simulink model "LGS_allFaultStuffDeleted"  (R2019b)
settings: Solver=FixedStepDiscrete  StartTime=0.0  StopTime=45.0  FixedStep=0.1  RelTol=1e-3
model workspace (MAT data in the model file):
  fipData : object (value not decoded)
  fipName : object (value not decoded)
  stepSize = 0.1
libraries: commrandsrc3 x16, simulink x3, LibFailureCondition x1
(part 2 of 7)

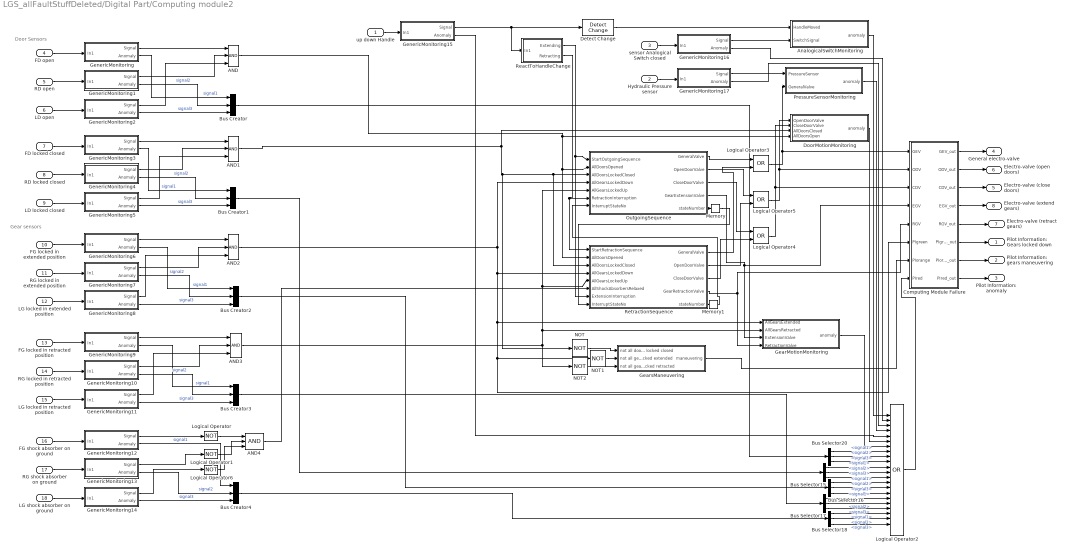
== system LGS_allFaultStuffDeleted/Digital Part/Computing module2 ==
  note: Gear sensors
  note: Door Sensors
  up down Handle : Inport
  Hydraulic Pressure sensor : Inport  Port=2
  " sensor Analogical Switch closed" : Inport  Port=3
  FD open : Inport  Port=4
  RD open : Inport  Port=5
  LD open : Inport  Port=6
  FD locked closed : Inport  Port=7
  RD locked closed : Inport  Port=8
  LD locked closed : Inport  Port=9
  FG locked in extended position : Inport  Port=10
  RG locked in extended position : Inport  Port=11
  LG locked in extended position : Inport  Port=12
  FG locked in retracted position : Inport  Port=13
  RG locked in retracted position : Inport  Port=14
  LG locked in retracted position : Inport  Port=15
  FG shock absorber on ground : Inport  Port=16
  RG shock absorber on ground : Inport  Port=17
  LG shock absorber on ground : Inport  Port=18
  AND{,1..4} (5 alike) : Logic  Inputs=3  IconShape=distinctive  AllPortsSameDT=off  OutDataTypeStr=boolean
  AnalogicalSwitchMonitoring : Stateflow chart  TreatAsAtomicUnit=on
  Bus Creator{,1..4} (5 alike) : BusCreator  Inputs=3
  Bus Selector{15..18,20} (5 alike) : BusSelector  OutputSignals=signal1,signal2,signal3
  Computing Module Failure : Subsystem
  Detect Change : simulink/Logic and Bit Operations/Detect Change  vinit=1  OutDataTypeStr=boolean
  DoorMotionMonitoring : Stateflow chart  TreatAsAtomicUnit=on
  GearMotionMonitoring : Stateflow chart  TreatAsAtomicUnit=on
  GearsManeuvering : Subsystem
  GenericMonitoring : Subsystem
  GenericMonitoring1 : Subsystem
  GenericMonitoring10 : Subsystem
  GenericMonitoring11 : Subsystem
  GenericMonitoring12 : Subsystem
  GenericMonitoring13 : Subsystem
  GenericMonitoring14 : Subsystem
  GenericMonitoring15 : Subsystem
  GenericMonitoring16 : Subsystem
  GenericMonitoring17 : Subsystem
  GenericMonitoring2 : Subsystem
  GenericMonitoring3 : Subsystem
  GenericMonitoring4 : Subsystem
  GenericMonitoring5 : Subsystem
  GenericMonitoring6 : Subsystem
  GenericMonitoring7 : Subsystem
  GenericMonitoring8 : Subsystem
  GenericMonitoring9 : Subsystem
  Logical Operator : Logic  Operator=NOT  AllPortsSameDT=off  OutDataTypeStr=boolean
  Logical Operator1 : Logic  Operator=NOT  AllPortsSameDT=off  OutDataTypeStr=boolean
  Logical Operator2 : Logic  Operator=OR  Inputs=22  AllPortsSameDT=off  OutDataTypeStr=boolean
  Logical Operator3 : Logic  Operator=OR  AllPortsSameDT=off  OutDataTypeStr=boolean
  Logical Operator4 : Logic  Operator=OR  AllPortsSameDT=off  OutDataTypeStr=boolean
  Logical Operator5 : Logic  Operator=OR  AllPortsSameDT=off  OutDataTypeStr=boolean
  Logical Operator6 : Logic  Operator=NOT  AllPortsSameDT=off  OutDataTypeStr=boolean
  Memory : Memory  InheritSampleTime=on
  Memory1 : Memory  InheritSampleTime=on
  NOT : Logic  Operator=NOT  IconShape=distinctive  AllPortsSameDT=off  OutDataTypeStr=boolean
  NOT1 : Logic  Operator=NOT  IconShape=distinctive  AllPortsSameDT=off  OutDataTypeStr=boolean
  NOT2 : Logic  Operator=NOT  IconShape=distinctive  AllPortsSameDT=off  OutDataTypeStr=boolean
  OutgoingSequence : Stateflow chart  TreatAsAtomicUnit=on
  PressureSensorMonitoring : Stateflow chart  TreatAsAtomicUnit=on
  ReactToHandleChange : Subsystem
  RetractionSequence : Stateflow chart  TreatAsAtomicUnit=on
  Pilot Information: Gears locked down : Outport  OutDataTypeStr=boolean
  Pilot Information: gears maneuvering : Outport  Port=2  OutDataTypeStr=boolean
  Pilot Information: anomaly : Outport  Port=3  OutDataTypeStr=boolean
  General electro-valve : Outport  Port=4
  Electro-valve (close doors) : Outport  Port=5
  Electro-valve (open doors) : Outport  Port=6
  Electro-valve (retract gears) : Outport  Port=7
  Electro-valve (extend gears) : Outport  Port=8
  wires:
  ReactToHandleChange/1(Extending) -> RetractionSequence/7(ExtensionInterruption), OutgoingSequence/1(StartOutgoingSequence)
  OutgoingSequence/1(GeneralValve) -> Logical Operator3/1
  OutgoingSequence/2(OpenDoorValve) -> Logical Operator5/1
  OutgoingSequence/4(GearExtensionValve) -> Computing Module Failure/4(EGV), GearMotionMonitoring/3(ExtensionValve)
  OutgoingSequence/3(CloseDoorValve) -> Logical Operator4/1
  FD open/1 -> GenericMonitoring/1(In1)
  RD open/1 -> GenericMonitoring1/1(In1)
  LD open/1 -> GenericMonitoring2/1(In1)
  AND/1 -> DoorMotionMonitoring/4(AllDoorsOpen), RetractionSequence/2(AllDoorsOpened), OutgoingSequence/2(AllDoorsOpened)
  FD locked closed/1 -> GenericMonitoring3/1(In1)
  RD locked closed/1 -> GenericMonitoring4/1(In1)
  LD locked closed/1 -> GenericMonitoring5/1(In1)
  AND1/1 -> NOT/1, RetractionSequence/3(AllDoorsLockedClosed), OutgoingSequence/3(AllDoorsLockedClosed), DoorMotionMonitoring/3(AllDoorsClosed)
  FG locked in extended position/1 -> GenericMonitoring6/1(In1)
  RG locked in extended position/1 -> GenericMonitoring7/1(In1)
  LG locked in extended position/1 -> GenericMonitoring8/1(In1)
  FG locked in retracted position/1 -> GenericMonitoring9/1(In1)
  RG locked in retracted position/1 -> GenericMonitoring10/1(In1)
  LG locked in retracted position/1 -> GenericMonitoring11/1(In1)
  LG shock absorber on ground/1 -> GenericMonitoring14/1(In1)
  AND2/1 -> Computing Module Failure/6(PIgreen), NOT1/1, GearMotionMonitoring/1(AllGearsExtended), RetractionSequence/4(AllGearsLockedDown), OutgoingSequence/4(AllGearsLockedDown)
  GearsManeuvering/1(maneuvering) -> Computing Module Failure/7(PIorange)
  FG shock absorber on ground/1 -> GenericMonitoring12/1(In1)
  GenericMonitoring12/1(Signal) -> Logical Operator/1
  GenericMonitoring13/1(Signal) -> Logical Operator1/1
  GenericMonitoring14/1(Signal) -> Logical Operator6/1
  AnalogicalSwitchMonitoring/1(anomaly) -> Logical Operator2/1
  Detect Change/1 -> AnalogicalSwitchMonitoring/1(HandleMoved)
  " sensor Analogical Switch closed"/1 -> GenericMonitoring16/1(In1)
  Hydraulic Pressure sensor/1 -> GenericMonitoring17/1(In1)
  PressureSensorMonitoring/1(anomaly) -> Logical Operator2/4
  DoorMotionMonitoring/1(anomaly) -> Logical Operator2/6
  GearMotionMonitoring/1(anomaly) -> Logical Operator2/7
  Logical Operator2/1 -> Computing Module Failure/8(PIred)
  RG shock absorber on ground/1 -> GenericMonitoring13/1(In1)
  RetractionSequence/1(GeneralValve) -> Logical Operator3/2
  Logical Operator3/1 -> Computing Module Failure/1(GEV), PressureSensorMonitoring/2(GeneralValve)
  RetractionSequence/3(CloseDoorValve) -> Logical Operator4/2
  Logical Operator4/1 -> Computing Module Failure/3(CDV), DoorMotionMonitoring/2(CloseDoorValve)
  RetractionSequence/2(OpenDoorValve) -> Logical Operator5/2
  Logical Operator5/1 -> Computing Module Failure/2(ODV), DoorMotionMonitoring/1(OpenDoorValve)
  RetractionSequence/4(GearRetractionValve) -> Computing Module Failure/5(RGV), GearMotionMonitoring/4(RetractionValve)
  GenericMonitoring/2(Anomaly) -> Bus Creator/1  "signal1"
  GenericMonitoring2/2(Anomaly) -> Bus Creator/3  "signal3"
  GenericMonitoring1/2(Anomaly) -> Bus Creator/2  "signal2"
  Bus Creator/1 -> Bus Selector20/1
  AND3/1 -> GearMotionMonitoring/2(AllGearsRetracted), RetractionSequence/5(AllGearsLockedUp), OutgoingSequence/5(AllGearsLockedUp), NOT2/1
  ReactToHandleChange/2(Retracting) -> RetractionSequence/1(StartRetractionSequence), OutgoingSequence/6(RetractionInterruption)
  Bus Selector15/1 -> Logical Operator2/11  "<signal1>"
  Bus Selector15/2 -> Logical Operator2/12  "<signal2>"
  Bus Selector15/3 -> Logical Operator2/13  "<signal3>"
  Bus Selector16/1 -> Logical Operator2/14  "<signal1>"
  Bus Selector16/2 -> Logical Operator2/15  "<signal2>"
  Bus Selector16/3 -> Logical Operator2/16  "<signal3>"
  Bus Selector17/1 -> Logical Operator2/17  "<signal1>"
  Bus Selector17/2 -> Logical Operator2/18  "<signal2>"
  Bus Selector17/3 -> Logical Operator2/19  "<signal3>"
  Bus Selector18/1 -> Logical Operator2/20  "<signal1>"
  Bus Selector18/2 -> Logical Operator2/21  "<signal2>"
  Bus Selector18/3 -> Logical Operator2/22  "<signal3>"
  Bus Selector20/1 -> Logical Operator2/8  "<signal1>"
  Bus Selector20/2 -> Logical Operator2/9  "<signal2>"
  Bus Selector20/3 -> Logical Operator2/10  "<signal3>"
  GenericMonitoring12/2(Anomaly) -> Bus Creator4/1  "signal1"
  GenericMonitoring3/2(Anomaly) -> Bus Creator1/1  "signal1"
  GenericMonitoring4/2(Anomaly) -> Bus Creator1/2  "signal2"
  GenericMonitoring5/2(Anomaly) -> Bus Creator1/3  "signal3"
  Bus Creator1/1 -> Bus Selector15/1
  GenericMonitoring8/2(Anomaly) -> Bus Creator2/3  "signal3"
  GenericMonitoring6/2(Anomaly) -> Bus Creator2/1  "signal1"
  GenericMonitoring7/2(Anomaly) -> Bus Creator2/2  "signal2"
  Bus Creator2/1 -> Bus Selector16/1
  GenericMonitoring11/2(Anomaly) -> Bus Creator3/3  "signal3"
  GenericMonitoring10/2(Anomaly) -> Bus Creator3/2  "signal2"
  GenericMonitoring9/2(Anomaly) -> Bus Creator3/1  "signal1"
  Bus Creator3/1 -> Bus Selector17/1
  GenericMonitoring13/2(Anomaly) -> Bus Creator4/2  "signal2"
  GenericMonitoring14/2(Anomaly) -> Bus Creator4/3  "signal3"
  Bus Creator4/1 -> Bus Selector18/1
  Logical Operator/1 -> AND4/1
  Logical Operator6/1 -> AND4/3
  GenericMonitoring17/1(Signal) -> PressureSensorMonitoring/1(PressureSensor)
  GenericMonitoring16/1(Signal) -> AnalogicalSwitchMonitoring/2(SwitchSignal)
  GenericMonitoring16/2(Anomaly) -> Logical Operator2/2
  up down Handle/1 -> GenericMonitoring15/1(In1)
  GenericMonitoring15/2(Anomaly) -> Logical Operator2/5
  GenericMonitoring17/2(Anomaly) -> Logical Operator2/3
  Memory/1 -> RetractionSequence/8(InterruptStateNo)
  Memory1/1 -> OutgoingSequence/7(InterruptStateNo)
  OutgoingSequence/5(stateNumber) -> Memory/1
  RetractionSequence/5(stateNumber) -> Memory1/1
  Computing Module Failure/1(GEV_out) -> General electro-valve/1
  Computing Module Failure/2(ODV_out) -> Electro-valve (open doors)/1
  Computing Module Failure/3(CDV_out) -> Electro-valve (close doors)/1
  Computing Module Failure/4(EGV_out) -> Electro-valve (extend gears)/1
  Computing Module Failure/5(RGV_out) -> Electro-valve (retract gears)/1
  Computing Module Failure/6(PIgreen_out) -> Pilot Information: Gears locked down/1
  Computing Module Failure/7(PIorange_out) -> Pilot Information: gears maneuvering/1
  Computing Module Failure/8(PIred_out) -> Pilot Information: anomaly/1
  AND4/1 -> RetractionSequence/6(AllShockAbsorbersRelaxed)
  GenericMonitoring15/1(Signal) -> Detect Change/1, ReactToHandleChange/1(In1)
  GenericMonitoring/1(Signal) -> AND/1
  GenericMonitoring1/1(Signal) -> AND/2
  GenericMonitoring2/1(Signal) -> AND/3
  GenericMonitoring3/1(Signal) -> AND1/1
  GenericMonitoring4/1(Signal) -> AND1/2
  GenericMonitoring5/1(Signal) -> AND1/3
  GenericMonitoring6/1(Signal) -> AND2/1
  GenericMonitoring7/1(Signal) -> AND2/2
  GenericMonitoring8/1(Signal) -> AND2/3
  GenericMonitoring9/1(Signal) -> AND3/1
  GenericMonitoring10/1(Signal) -> AND3/2
  GenericMonitoring11/1(Signal) -> AND3/3
  NOT/1 -> GearsManeuvering/1(not all doors locked closed)
  NOT1/1 -> GearsManeuvering/2(not all gears locked extended)
  NOT2/1 -> GearsManeuvering/3(not all gears locked retracted)
  Logical Operator1/1 -> AND4/2

== system LGS_allFaultStuffDeleted/Doors/EV close doors ==
  In1 : Inport
  In2 : Inport  Port=2
  Constant : Constant  Value=false  OutDataTypeStr=boolean
  EV close doors : Stateflow chart  TreatAsAtomicUnit=on
  Memory : Memory  InheritSampleTime=on
  Out1 : Outport
  wires:
  Memory/1 -> EV close doors/1(signal_in)
  In1/1 -> Memory/1
  In2/1 -> EV close doors/2(EVCloseDoorsPresure_in)
  EV close doors/1(EVCloseDoorsPresure_out) -> Out1/1
  Constant/1 -> EV close doors/3(fail)

== system LGS_allFaultStuffDeleted/Doors/EV open doors ==
  In1 : Inport
  In2 : Inport  Port=2
  Constant : Constant  Value=false  OutDataTypeStr=boolean
  EV open doors : Stateflow chart  TreatAsAtomicUnit=on
  Memory1 : Memory  InheritSampleTime=on
  Out1 : Outport
  wires:
  Memory1/1 -> EV open doors/1(signal_in)
  In1/1 -> Memory1/1
  In2/1 -> EV open doors/2(EVOpenDoorsPresure_in)
  Constant/1 -> EV open doors/3(fail)
  EV open doors/1(EVOpenDoorsPresure_out) -> Out1/1

== system LGS_allFaultStuffDeleted/Doors/front door zylinder ==
  note: [true, false]
  note: [true, false]
  presure open door : Inport  OutDataTypeStr=boolean
  presure close door : Inport  Port=2  OutDataTypeStr=boolean
  Constant : Constant  Value=false  OutDataTypeStr=boolean
  door cylinder : Stateflow chart  TreatAsAtomicUnit=on
  sensor locked closed : Subsystem
  sensor open : Subsystem
  sensor locked closed output : Outport
  sensor open output : Outport  Port=2
  door locked closed : Outport  Port=3
  wires:
  sensor open/1(sensor output) -> sensor open output/1
  sensor locked closed/1(sensor output) -> sensor locked closed output/1
  door cylinder/1(doorZylinderLockedClosed) -> door locked closed/1, sensor locked closed/1(sensor input)
  door cylinder/2(doorZylinderOpen) -> sensor open/1(sensor input)
  presure open door/1 -> door cylinder/1(presureOpenDoor)
  presure close door/1 -> door cylinder/2(presureCloseDoor)
  Constant/1 -> door cylinder/3(fail)

== system LGS_allFaultStuffDeleted/Doors/left door zylinder ==
  note: [true, false]
  note: [true, false]
  presure open door : Inport  OutDataTypeStr=boolean
  presure close door : Inport  Port=2  OutDataTypeStr=boolean
  Constant : Constant  Value=false  OutDataTypeStr=boolean
  door zylinder : Stateflow chart  TreatAsAtomicUnit=on
  sensor locked closed : Subsystem
  sensor open : Subsystem
  sensor locked closed output : Outport
  sensor open output : Outport  Port=2
  door locked closed : Outport  Port=3
  wires:
  Constant/1 -> door zylinder/3(fail)
  sensor open/1(sensor output) -> sensor open output/1
  sensor locked closed/1(sensor output) -> sensor locked closed output/1
  door zylinder/2(doorZylinderOpen) -> sensor open/1(sensor input)
  presure open door/1 -> door zylinder/1(presureOpenDoor)
  presure close door/1 -> door zylinder/2(presureCloseDoor)
  door zylinder/1(doorZylinderLockedClosed) -> door locked closed/1, sensor locked closed/1(sensor input)

== system LGS_allFaultStuffDeleted/Doors/right door zylinder ==
  note: [true, false]
  note: [true, false]
  presure open door : Inport  OutDataTypeStr=boolean
  presure close door : Inport  Port=2  OutDataTypeStr=boolean
  Constant : Constant  Value=false  OutDataTypeStr=boolean
  door zylinder : Stateflow chart  TreatAsAtomicUnit=on
  sensor locked closed : Subsystem
  sensor open : Subsystem
  sensor locked closed output : Outport
  sensor open output : Outport  Port=2
  door locked closed : Outport  Port=3
  wires:
  Constant/1 -> door zylinder/3(fail)
  sensor open/1(sensor output) -> sensor open output/1
  sensor locked closed/1(sensor output) -> sensor locked closed output/1
  door zylinder/2(doorZylinderOpen) -> sensor open/1(sensor input)
  presure open door/1 -> door zylinder/1(presureOpenDoor)
  presure close door/1 -> door zylinder/2(presureCloseDoor)
  door zylinder/1(doorZylinderLockedClosed) -> door locked closed/1, sensor locked closed/1(sensor input)

== system LGS_allFaultStuffDeleted/FailureConditionObserver/FC1 ==
  Retraction Valve : Inport
  Extension Valve : Inport  Port=2
  ActualSystemCondition : Subsystem  AncestorBlock=LibFailureCondition/ActualSystemCondition  mask(ActualSystemCondition){}
      mask help: ActualSystemCondition
      mask Help: ActualSystemCondition
  FC1 : Terminator  mask(DiveObserver){}
      mask help: DiveObserver
      settings: AncestorBlock=LibFailureCondition/DiveObserver
      mask Help: DiveObserver
      mask Display: image('icons/observer.png','center')
  FC_FC1_output : Subsystem  AncestorBlock=LibFailureCondition/ExpectedSystemBehavior  mask(ExpectedSystemBehavior){}
      mask help: ExpectedSystemBehavior
      mask Help: ExpectedSystemBehavior
  wires:
  ActualSystemCondition/1("Activate Observer ") -> FC_FC1_output/1(ActivateObserver)
  FC_FC1_output/1(ConditionState) -> FC1/1
  Retraction Valve/1 -> FC_FC1_output/2(Retraction Valve)
  Extension Valve/1 -> FC_FC1_output/3(Extension Valve)

== system LGS_allFaultStuffDeleted/FailureConditionObserver/FC2 ==
  Red LED : Inport
  FG locked extended : Inport  Port=2
  "LG locked extended " : Inport  Port=3
  RG locked extended : Inport  Port=4
  FD locked closed : Inport  Port=5
  LD locked closed : Inport  Port=6
  RD locked closed : Inport  Port=7
  Command Handle : Inport  Port=8
  ActualSystemCondition : Subsystem  AncestorBlock=LibFailureCondition/ActualSystemCondition  mask(ActualSystemCondition){}
      mask help: ActualSystemCondition
      mask Help: ActualSystemCondition
  FC2 : Terminator  mask(DiveObserver){}
      mask help: DiveObserver
      settings: AncestorBlock=LibFailureCondition/DiveObserver
      mask Help: DiveObserver
      mask Display: image('icons/observer.png','center')
  FC_FC2_output : Subsystem  AncestorBlock=LibFailureCondition/ExpectedSystemBehavior  mask(ExpectedSystemBehavior){}
      mask help: ExpectedSystemBehavior
      mask Help: ExpectedSystemBehavior
  wires:
  FC_FC2_output/1(ConditionState) -> FC2/1
  ActualSystemCondition/1("Activate Observer ") -> FC_FC2_output/1(ActivateObserver)
  Red LED/1 -> FC_FC2_output/9(Red LED)
  FG locked extended/1 -> FC_FC2_output/3(FG locked down)
  RG locked extended/1 -> FC_FC2_output/4(RG locked down)
  RD locked closed/1 -> FC_FC2_output/7(RD locked closed)
  FD locked closed/1 -> FC_FC2_output/6(FD locked closed)
  LD locked closed/1 -> FC_FC2_output/8(LD locked closed)
  Command Handle/1 -> FC_FC2_output/2(Command Handle)
  "LG locked extended "/1 -> FC_FC2_output/5(LG locked down)

== system LGS_allFaultStuffDeleted/FailureConditionObserver/FC3 ==
  Green LED : Inport
  Orange LED : Inport  Port=2
  Red LED : Inport  Port=3
  FG locked extended : Inport  Port=4
  LG locked extended : Inport  Port=5
  RG locked extended : Inport  Port=6
  FD locked closed : Inport  Port=7
  LD locked closed : Inport  Port=8
  RD locked closed : Inport  Port=9
  ActualSystemCondition : Subsystem  AncestorBlock=LibFailureCondition/ActualSystemCondition  mask(ActualSystemCondition){}
      mask help: ActualSystemCondition
      mask Help: ActualSystemCondition
  FC3 : LibFailureCondition/DiveObserver
      settings: SourceProductName=Failure Condition
  FC_FC3_output : Subsystem  AncestorBlock=LibFailureCondition/ExpectedSystemBehavior  mask(ExpectedSystemBehavior){}
      mask help: ExpectedSystemBehavior
      mask Help: ExpectedSystemBehavior
  wires:
  FC_FC3_output/1(ConditionState) -> FC3/1
  ActualSystemCondition/1("Activate Observer ") -> FC_FC3_output/1(ActivateObserver)
  Green LED/1 -> ActualSystemCondition/1(Green LED)
  Orange LED/1 -> ActualSystemCondition/2(Orange LED)
  Red LED/1 -> ActualSystemCondition/3(Red LED)
  FG locked extended/1 -> FC_FC3_output/2(FG locked down)
  LG locked extended/1 -> FC_FC3_output/4(LG locked down)
  RG locked extended/1 -> FC_FC3_output/3(RG locked down)
  FD locked closed/1 -> FC_FC3_output/5(FD locked closed1)
  LD locked closed/1 -> FC_FC3_output/7(LD locked closed1)
  RD locked closed/1 -> FC_FC3_output/6(RD locked closed1)

== system LGS_allFaultStuffDeleted/Gears/EV extend gear ==
  In1 : Inport
  In2 : Inport  Port=2
  Constant : Constant  Value=false  OutDataTypeStr=boolean
  EV extend gear : Stateflow chart  TreatAsAtomicUnit=on
  Memory : Memory  InheritSampleTime=on
  Out1 : Outport
  wires:
  Memory/1 -> EV extend gear/1(signal_in)
  In1/1 -> Memory/1
  In2/1 -> EV extend gear/2(EVExtendGearPresure_in)
  Constant/1 -> EV extend gear/3(fail)
  EV extend gear/1(EVExtendGearPresure_out) -> Out1/1

== system LGS_allFaultStuffDeleted/Gears/EV retract gear ==
  In1 : Inport
  In2 : Inport  Port=2
  Constant : Constant  Value=false  OutDataTypeStr=boolean
  EV retract gear : Stateflow chart  TreatAsAtomicUnit=on
  Memory1 : Memory  InheritSampleTime=on
  Out1 : Outport
  wires:
  Memory1/1 -> EV retract gear/1(signal_in)
  In1/1 -> Memory1/1
  In2/1 -> EV retract gear/2(EVRetractGearPresure_in)
  Constant/1 -> EV retract gear/3(fail)
  EV retract gear/1(EVRetractGearPresure_out) -> Out1/1

== system LGS_allFaultStuffDeleted/Gears/FG shock absorber ==
  shock absorber in : Inport  OutDataTypeStr=boolean
  sensor shock absorber : Subsystem
  sensor shock absorber output : Outport
  wires:
  shock absorber in/1 -> sensor shock absorber/1(sensor input)
  sensor shock absorber/1(sensor output) -> sensor shock absorber output/1

== system LGS_allFaultStuffDeleted/Gears/LG shock absorber ==
  shock absorber in : Inport  OutDataTypeStr=boolean
  sensor shock absorber : Subsystem
  sensor shock absorber output : Outport
  wires:
  shock absorber in/1 -> sensor shock absorber/1(sensor input)
  sensor shock absorber/1(sensor output) -> sensor shock absorber output/1

== system LGS_allFaultStuffDeleted/Gears/RG shock absorber ==
  shock absorber in : Inport  OutDataTypeStr=boolean
  sensor shock absorber : Subsystem
  sensor shock absorber output : Outport
  wires:
  shock absorber in/1 -> sensor shock absorber/1(sensor input)
  sensor shock absorber/1(sensor output) -> sensor shock absorber output/1

== system LGS_allFaultStuffDeleted/Gears/front gear cylinder ==
  note: [true, false]
  note: [true, false]
  presure extend gear : Inport  OutDataTypeStr=boolean
  presure retract gear : Inport  Port=2  OutDataTypeStr=boolean
  initial handle state : Inport  Port=3
  Constant : Constant  Value=false  OutDataTypeStr=boolean
  gear zylinder : Stateflow chart  TreatAsAtomicUnit=on
  sensor locked extended : Subsystem
  sensor locked retracted : Subsystem
  sensor locked extended output : Outport
  sensor locked retracted output : Outport  Port=2
  gear locked extended : Outport  Port=3
  gear locked retracted : Outport  Port=4
  wires:
  Constant/1 -> gear zylinder/3(fail)
  presure retract gear/1 -> gear zylinder/2(presureRetractGear)
  presure extend gear/1 -> gear zylinder/1(presureExtendGear)
  gear zylinder/1(gearLockedExtended) -> gear locked extended/1, sensor locked extended/1(sensor input)
  sensor locked extended/1(sensor output) -> sensor locked extended output/1
  gear zylinder/2(gearLockedRetracted) -> gear locked retracted/1, sensor locked retracted/1(sensor input)
  sensor locked retracted/1(sensor output) -> sensor locked retracted output/1
  initial handle state/1 -> gear zylinder/4(initHandleState)

== system LGS_allFaultStuffDeleted/Gears/left gear cylinder ==
  note: [true, false]
  note: [true, false]
  presure extend gear : Inport  OutDataTypeStr=boolean
  presure retract gear : Inport  Port=2  OutDataTypeStr=boolean
  initial handle state : Inport  Port=3
  Constant : Constant  Value=false  OutDataTypeStr=boolean
  gear zylinder : Stateflow chart  TreatAsAtomicUnit=on
  sensor locked extended : Subsystem
  sensor locked retracted : Subsystem
  sensor locked extended output : Outport
  sensor locked retracted output : Outport  Port=2
  gear locked extended : Outport  Port=3
  gear locked retracted : Outport  Port=4
  wires:
  Constant/1 -> gear zylinder/3(fail)
  presure retract gear/1 -> gear zylinder/2(presureRetractGear)
  presure extend gear/1 -> gear zylinder/1(presureExtendGear)
  sensor locked extended/1(sensor output) -> sensor locked extended output/1
  sensor locked retracted/1(sensor output) -> sensor locked retracted output/1
  gear zylinder/1(gearLockedExtended) -> gear locked extended/1, sensor locked extended/1(sensor input)
  gear zylinder/2(gearLockedRetracted) -> gear locked retracted/1, sensor locked retracted/1(sensor input)
  initial handle state/1 -> gear zylinder/4(initHandleState)

== system LGS_allFaultStuffDeleted/Gears/right gear cylinder ==
  note: [true, false]
  note: [true, false]
  presure extend gear : Inport  OutDataTypeStr=boolean
  presure retract gear : Inport  Port=2  OutDataTypeStr=boolean
  initial handle state : Inport  Port=3
  Constant : Constant  Value=false  OutDataTypeStr=boolean
  gear zylinder : Stateflow chart  TreatAsAtomicUnit=on
  sensor locked extended : Subsystem
  sensor locked retracted : Subsystem
  sensor locked extended output : Outport
  sensor locked retracted output : Outport  Port=2
  gear locked extended : Outport  Port=3
  gear locked retracted : Outport  Port=4
  wires:
  Constant/1 -> gear zylinder/3(fail)
  presure retract gear/1 -> gear zylinder/2(presureRetractGear)
  presure extend gear/1 -> gear zylinder/1(presureExtendGear)
  sensor locked extended/1(sensor output) -> sensor locked extended output/1
  sensor locked retracted/1(sensor output) -> sensor locked retracted output/1
  gear zylinder/1(gearLockedExtended) -> gear locked extended/1, sensor locked extended/1(sensor input)
  gear zylinder/2(gearLockedRetracted) -> gear locked retracted/1, sensor locked retracted/1(sensor input)
  initial handle state/1 -> gear zylinder/4(initHandleState)

== system LGS_allFaultStuffDeleted/sensor up down handle/FIP1 ==
  In1 : Inport
  Out1 : Outport
  wires:
  In1/1 -> Out1/1

== system LGS_allFaultStuffDeleted/sensor up down handle/FIP2 ==
  In1 : Inport
  Out1 : Outport
  wires:
  In1/1 -> Out1/1

== system LGS_allFaultStuffDeleted/sensor up down handle/FIP3 ==
  In1 : Inport
  Out1 : Outport
  wires:
  In1/1 -> Out1/1

== system LGS_allFaultStuffDeleted/Analogical switch and general electro-valve and pressure sensor/sensor switch closed/FIP1 ==
  In1 : Inport
  Out1 : Outport
  wires:
  In1/1 -> Out1/1

== system LGS_allFaultStuffDeleted/Analogical switch and general electro-valve and pressure sensor/sensor switch closed/FIP2 ==
  In1 : Inport
  Out1 : Outport
  wires:
  In1/1 -> Out1/1

== system LGS_allFaultStuffDeleted/Analogical switch and general electro-valve and pressure sensor/sensor switch closed/FIP3 ==
  In1 : Inport
  Out1 : Outport
  wires:
  In1/1 -> Out1/1

== system LGS_allFaultStuffDeleted/Analogical switch and general electro-valve and pressure sensor/sensor system pressurized/FIP1 ==
  In1 : Inport
  Out1 : Outport
  wires:
  In1/1 -> Out1/1

== system LGS_allFaultStuffDeleted/Analogical switch and general electro-valve and pressure sensor/sensor system pressurized/FIP2 ==
  In1 : Inport
  Out1 : Outport
  wires:
  In1/1 -> Out1/1

== system LGS_allFaultStuffDeleted/Analogical switch and general electro-valve and pressure sensor/sensor system pressurized/FIP3 ==
  In1 : Inport
  Out1 : Outport
  wires:
  In1/1 -> Out1/1

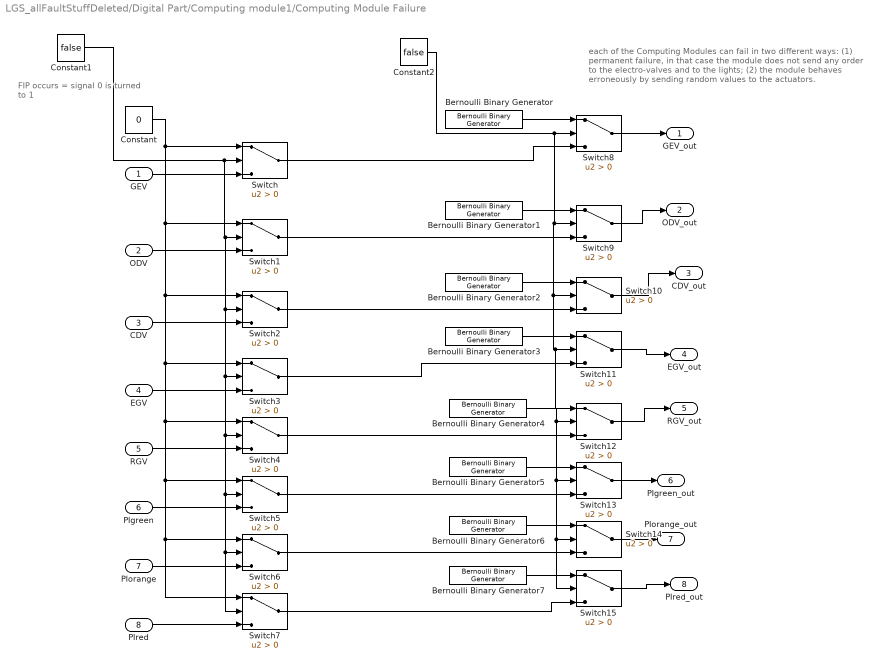
== system LGS_allFaultStuffDeleted/Digital Part/Computing module1/Computing Module Failure ==
  note: FIP occurs = signal 0
      | is turned to 1
  note: each of the Computing Modules can fail in two different ways: (1) permanent failure, in that case the module does not send any order to the electro-valves and to the lights;
      | (2) the module behaves erroneously by sending random values to the actuators.
  GEV : Inport
  ODV : Inport  Port=2
  CDV : Inport  Port=3
  EGV : Inport  Port=4
  RGV : Inport  Port=5
  PIgreen : Inport  Port=6
  PIorange : Inport  Port=7
  PIred : Inport  Port=8
  Bernoulli Binary Generator{,1..7} (8 alike) : commrandsrc3/Bernoulli Binary Generator  ProbabilityOfZero=0.5  SeedSource=Auto  Seed=0  SampleTime=-1  SamplesPerFrame=1  OutputDataType=boolean  SimulateUsing=Interpreted execution
      settings: SourceProductName=Communications Toolbox
  Constant : Constant  Value=0  OutDataTypeStr=boolean
  Constant1 : Constant  Value=false  OutDataTypeStr=boolean
  Constant2 : Constant  Value=false  OutDataTypeStr=boolean
  Switch{,1..15} (16 alike) : Switch  Criteria=u2 > Threshold
  GEV_out : Outport
  ODV_out : Outport  Port=2
  CDV_out : Outport  Port=3
  EGV_out : Outport  Port=4
  RGV_out : Outport  Port=5
  PIgreen_out : Outport  Port=6
  PIorange_out : Outport  Port=7
  PIred_out : Outport  Port=8
  wires:
  Constant/1 -> Switch4/1, Switch7/1, Switch6/1, Switch5/1, Switch3/1, Switch2/1, Switch1/1, Switch/1
  Constant1/1 -> Switch4/2, Switch7/2, Switch6/2, Switch5/2, Switch3/2, Switch2/2, Switch1/2, Switch/2
  GEV/1 -> Switch/3
  ODV/1 -> Switch1/3
  CDV/1 -> Switch2/3
  EGV/1 -> Switch3/3
  RGV/1 -> Switch4/3
  PIgreen/1 -> Switch5/3
  PIorange/1 -> Switch6/3
  PIred/1 -> Switch7/3
  Bernoulli Binary Generator/1 -> Switch8/1
  Constant2/1 -> Switch8/2, Switch15/2, Switch14/2, Switch13/2, Switch12/2, Switch11/2, Switch10/2, Switch9/2
  Switch/1 -> Switch8/3
  Switch1/1 -> Switch9/3
  Switch2/1 -> Switch10/3
  Switch3/1 -> Switch11/3
  Switch4/1 -> Switch12/3
  Switch5/1 -> Switch13/3
  Switch6/1 -> Switch14/3
  Switch7/1 -> Switch15/3
  Switch8/1 -> GEV_out/1
  Switch9/1 -> ODV_out/1
  Switch10/1 -> CDV_out/1
  Switch11/1 -> EGV_out/1
  Switch12/1 -> RGV_out/1
  Switch13/1 -> PIgreen_out/1
  Switch14/1 -> PIorange_out/1
  Switch15/1 -> PIred_out/1
  Bernoulli Binary Generator1/1 -> Switch9/1
  Bernoulli Binary Generator2/1 -> Switch10/1
  Bernoulli Binary Generator3/1 -> Switch11/1
  Bernoulli Binary Generator4/1 -> Switch12/1
  Bernoulli Binary Generator5/1 -> Switch13/1
  Bernoulli Binary Generator6/1 -> Switch14/1
  Bernoulli Binary Generator7/1 -> Switch15/1

== system LGS_allFaultStuffDeleted/Digital Part/Computing module1/GearsManeuvering ==
  not all doors locked closed : Inport
  not all gears locked extended : Inport  Port=2
  not all gears locked retracted : Inport  Port=3
  Logical Operator : Logic  Operator=OR  AllPortsSameDT=off  OutDataTypeStr=boolean
  Logical Operator1 : Logic  AllPortsSameDT=off  OutDataTypeStr=boolean
  maneuvering : Outport
  wires:
  not all doors locked closed/1 -> Logical Operator/1
  not all gears locked extended/1 -> Logical Operator1/1
  not all gears locked retracted/1 -> Logical Operator1/2
  Logical Operator/1 -> maneuvering/1
  Logical Operator1/1 -> Logical Operator/2

== system LGS_allFaultStuffDeleted/Digital Part/Computing module1/GenericMonitoring ==
  In1 : Inport
  AND : Logic  Inputs=3  IconShape=distinctive  AllPortsSameDT=off  OutDataTypeStr=boolean
  Bus Selector : BusSelector  OutputSignals=signal1,signal2,signal3
  GenericMonitoring2 : Stateflow chart  TreatAsAtomicUnit=on
  Logical Operator1 : Logic  Operator=XOR  AllPortsSameDT=off  OutDataTypeStr=boolean
  Logical Operator2 : Logic  Operator=XOR  AllPortsSameDT=off  OutDataTypeStr=boolean
  Logical Operator3 : Logic  Operator=NOT  AllPortsSameDT=off  OutDataTypeStr=boolean
  Logical Operator4 : Logic  Operator=NOT  AllPortsSameDT=off  OutDataTypeStr=boolean
  Switch : Switch  Criteria=u2 > Threshold
  Switch1 : Switch  Criteria=u2 > Threshold
  Switch2 : Switch  Criteria=u2 > Threshold
  Signal : Outport  OutDataTypeStr=boolean
  Anomaly : Outport  Port=2  OutDataTypeStr=boolean
  wires:
  Bus Selector/1 -> GenericMonitoring2/1(Channel1), Logical Operator1/1, Switch1/1, Switch/1, AND/1  "<signal1>"
  Bus Selector/2 -> AND/2, GenericMonitoring2/2(Channel2), Logical Operator1/2, Logical Operator2/1, Switch2/1  "<signal2>"
  Bus Selector/3 -> AND/3, GenericMonitoring2/3(Channel3), Logical Operator2/2, Switch2/3  "<signal3>"
  In1/1 -> Bus Selector/1
  AND/1 -> Switch/2
  GenericMonitoring2/1(anomaly) -> Anomaly/1
  Switch/1 -> Signal/1
  Logical Operator4/1 -> Switch1/2
  Logical Operator2/1 -> Logical Operator3/1
  Switch2/1 -> Switch1/3
  Switch1/1 -> Switch/3
  Logical Operator3/1 -> Switch2/2
  Logical Operator1/1 -> Logical Operator4/1

== system LGS_allFaultStuffDeleted/Digital Part/Computing module1/GenericMonitoring1 ==
  In1 : Inport
  AND : Logic  Inputs=3  IconShape=distinctive  AllPortsSameDT=off  OutDataTypeStr=boolean
  Bus Selector : BusSelector  OutputSignals=signal1,signal2,signal3
  GenericMonitoring2 : Stateflow chart  TreatAsAtomicUnit=on
  Logical Operator1 : Logic  Operator=XOR  AllPortsSameDT=off  OutDataTypeStr=boolean
  Logical Operator2 : Logic  Operator=XOR  AllPortsSameDT=off  OutDataTypeStr=boolean
  Logical Operator3 : Logic  Operator=NOT  AllPortsSameDT=off  OutDataTypeStr=boolean
  Logical Operator4 : Logic  Operator=NOT  AllPortsSameDT=off  OutDataTypeStr=boolean
  Switch : Switch  Criteria=u2 > Threshold
  Switch1 : Switch  Criteria=u2 > Threshold
  Switch2 : Switch  Criteria=u2 > Threshold
  Signal : Outport  OutDataTypeStr=boolean
  Anomaly : Outport  Port=2  OutDataTypeStr=boolean
  wires:
  Bus Selector/1 -> GenericMonitoring2/1(Channel1), Logical Operator1/1, Switch1/1, Switch/1, AND/1  "<signal1>"
  Bus Selector/2 -> AND/2, GenericMonitoring2/2(Channel2), Logical Operator1/2, Logical Operator2/1, Switch2/1  "<signal2>"
  Bus Selector/3 -> AND/3, GenericMonitoring2/3(Channel3), Logical Operator2/2, Switch2/3  "<signal3>"
  In1/1 -> Bus Selector/1
  AND/1 -> Switch/2
  GenericMonitoring2/1(anomaly) -> Anomaly/1
  Switch/1 -> Signal/1
  Logical Operator4/1 -> Switch1/2
  Logical Operator2/1 -> Logical Operator3/1
  Switch2/1 -> Switch1/3
  Switch1/1 -> Switch/3
  Logical Operator3/1 -> Switch2/2
  Logical Operator1/1 -> Logical Operator4/1

== system LGS_allFaultStuffDeleted/Digital Part/Computing module1/GenericMonitoring10 ==
  In1 : Inport
  AND : Logic  Inputs=3  IconShape=distinctive  AllPortsSameDT=off  OutDataTypeStr=boolean
  Bus Selector : BusSelector  OutputSignals=signal1,signal2,signal3
  GenericMonitoring2 : Stateflow chart  TreatAsAtomicUnit=on
  Logical Operator1 : Logic  Operator=XOR  AllPortsSameDT=off  OutDataTypeStr=boolean
  Logical Operator2 : Logic  Operator=XOR  AllPortsSameDT=off  OutDataTypeStr=boolean
  Logical Operator3 : Logic  Operator=NOT  AllPortsSameDT=off  OutDataTypeStr=boolean
  Logical Operator4 : Logic  Operator=NOT  AllPortsSameDT=off  OutDataTypeStr=boolean
  Switch : Switch  Criteria=u2 > Threshold
  Switch1 : Switch  Criteria=u2 > Threshold
  Switch2 : Switch  Criteria=u2 > Threshold
  Signal : Outport  OutDataTypeStr=boolean
  Anomaly : Outport  Port=2  OutDataTypeStr=boolean
  wires:
  Bus Selector/1 -> GenericMonitoring2/1(Channel1), Logical Operator1/1, Switch1/1, Switch/1, AND/1  "<signal1>"
  Bus Selector/2 -> AND/2, GenericMonitoring2/2(Channel2), Logical Operator1/2, Logical Operator2/1, Switch2/1  "<signal2>"
  Bus Selector/3 -> AND/3, GenericMonitoring2/3(Channel3), Logical Operator2/2, Switch2/3  "<signal3>"
  In1/1 -> Bus Selector/1
  AND/1 -> Switch/2
  GenericMonitoring2/1(anomaly) -> Anomaly/1
  Switch/1 -> Signal/1
  Logical Operator4/1 -> Switch1/2
  Logical Operator2/1 -> Logical Operator3/1
  Switch2/1 -> Switch1/3
  Switch1/1 -> Switch/3
  Logical Operator3/1 -> Switch2/2
  Logical Operator1/1 -> Logical Operator4/1

== system LGS_allFaultStuffDeleted/Digital Part/Computing module1/GenericMonitoring11 ==
  In1 : Inport
  AND : Logic  Inputs=3  IconShape=distinctive  AllPortsSameDT=off  OutDataTypeStr=boolean
  Bus Selector : BusSelector  OutputSignals=signal1,signal2,signal3
  GenericMonitoring2 : Stateflow chart  TreatAsAtomicUnit=on
  Logical Operator1 : Logic  Operator=XOR  AllPortsSameDT=off  OutDataTypeStr=boolean
  Logical Operator2 : Logic  Operator=XOR  AllPortsSameDT=off  OutDataTypeStr=boolean
  Logical Operator3 : Logic  Operator=NOT  AllPortsSameDT=off  OutDataTypeStr=boolean
  Logical Operator4 : Logic  Operator=NOT  AllPortsSameDT=off  OutDataTypeStr=boolean
  Switch : Switch  Criteria=u2 > Threshold
  Switch1 : Switch  Criteria=u2 > Threshold
  Switch2 : Switch  Criteria=u2 > Threshold
  Signal : Outport  OutDataTypeStr=boolean
  Anomaly : Outport  Port=2  OutDataTypeStr=boolean
  wires:
  Bus Selector/1 -> GenericMonitoring2/1(Channel1), Logical Operator1/1, Switch1/1, Switch/1, AND/1  "<signal1>"
  Bus Selector/2 -> AND/2, GenericMonitoring2/2(Channel2), Logical Operator1/2, Logical Operator2/1, Switch2/1  "<signal2>"
  Bus Selector/3 -> AND/3, GenericMonitoring2/3(Channel3), Logical Operator2/2, Switch2/3  "<signal3>"
  In1/1 -> Bus Selector/1
  AND/1 -> Switch/2
  GenericMonitoring2/1(anomaly) -> Anomaly/1
  Switch/1 -> Signal/1
  Logical Operator4/1 -> Switch1/2
  Logical Operator2/1 -> Logical Operator3/1
  Switch2/1 -> Switch1/3
  Switch1/1 -> Switch/3
  Logical Operator3/1 -> Switch2/2
  Logical Operator1/1 -> Logical Operator4/1

== system LGS_allFaultStuffDeleted/Digital Part/Computing module1/GenericMonitoring12 ==
  In1 : Inport
  AND : Logic  Inputs=3  IconShape=distinctive  AllPortsSameDT=off  OutDataTypeStr=boolean
  Bus Selector : BusSelector  OutputSignals=signal1,signal2,signal3
  GenericMonitoring2 : Stateflow chart  TreatAsAtomicUnit=on
  Logical Operator1 : Logic  Operator=XOR  AllPortsSameDT=off  OutDataTypeStr=boolean
  Logical Operator2 : Logic  Operator=XOR  AllPortsSameDT=off  OutDataTypeStr=boolean
  Logical Operator3 : Logic  Operator=NOT  AllPortsSameDT=off  OutDataTypeStr=boolean
  Logical Operator4 : Logic  Operator=NOT  AllPortsSameDT=off  OutDataTypeStr=boolean
  Switch : Switch  Criteria=u2 > Threshold
  Switch1 : Switch  Criteria=u2 > Threshold
  Switch2 : Switch  Criteria=u2 > Threshold
  Signal : Outport  OutDataTypeStr=boolean
  Anomaly : Outport  Port=2  OutDataTypeStr=boolean
  wires:
  Bus Selector/1 -> GenericMonitoring2/1(Channel1), Logical Operator1/1, Switch1/1, Switch/1, AND/1  "<signal1>"
  Bus Selector/2 -> AND/2, GenericMonitoring2/2(Channel2), Logical Operator1/2, Logical Operator2/1, Switch2/1  "<signal2>"
  Bus Selector/3 -> AND/3, GenericMonitoring2/3(Channel3), Logical Operator2/2, Switch2/3  "<signal3>"
  In1/1 -> Bus Selector/1
  AND/1 -> Switch/2
  GenericMonitoring2/1(anomaly) -> Anomaly/1
  Switch/1 -> Signal/1
  Logical Operator4/1 -> Switch1/2
  Logical Operator2/1 -> Logical Operator3/1
  Switch2/1 -> Switch1/3
  Switch1/1 -> Switch/3
  Logical Operator3/1 -> Switch2/2
  Logical Operator1/1 -> Logical Operator4/1

== system LGS_allFaultStuffDeleted/Digital Part/Computing module1/GenericMonitoring13 ==
  In1 : Inport
  AND : Logic  Inputs=3  IconShape=distinctive  AllPortsSameDT=off  OutDataTypeStr=boolean
  Bus Selector : BusSelector  OutputSignals=signal1,signal2,signal3
  GenericMonitoring2 : Stateflow chart  TreatAsAtomicUnit=on
  Logical Operator1 : Logic  Operator=XOR  AllPortsSameDT=off  OutDataTypeStr=boolean
  Logical Operator2 : Logic  Operator=XOR  AllPortsSameDT=off  OutDataTypeStr=boolean
  Logical Operator3 : Logic  Operator=NOT  AllPortsSameDT=off  OutDataTypeStr=boolean
  Logical Operator4 : Logic  Operator=NOT  AllPortsSameDT=off  OutDataTypeStr=boolean
  Switch : Switch  Criteria=u2 > Threshold
  Switch1 : Switch  Criteria=u2 > Threshold
  Switch2 : Switch  Criteria=u2 > Threshold
  Signal : Outport  OutDataTypeStr=boolean
  Anomaly : Outport  Port=2  OutDataTypeStr=boolean
  wires:
  Bus Selector/1 -> GenericMonitoring2/1(Channel1), Logical Operator1/1, Switch1/1, Switch/1, AND/1  "<signal1>"
  Bus Selector/2 -> AND/2, GenericMonitoring2/2(Channel2), Logical Operator1/2, Logical Operator2/1, Switch2/1  "<signal2>"
  Bus Selector/3 -> AND/3, GenericMonitoring2/3(Channel3), Logical Operator2/2, Switch2/3  "<signal3>"
  In1/1 -> Bus Selector/1
  AND/1 -> Switch/2
  GenericMonitoring2/1(anomaly) -> Anomaly/1
  Switch/1 -> Signal/1
  Logical Operator4/1 -> Switch1/2
  Logical Operator2/1 -> Logical Operator3/1
  Switch2/1 -> Switch1/3
  Switch1/1 -> Switch/3
  Logical Operator3/1 -> Switch2/2
  Logical Operator1/1 -> Logical Operator4/1

== system LGS_allFaultStuffDeleted/Digital Part/Computing module1/GenericMonitoring14 ==
  In1 : Inport
  AND : Logic  Inputs=3  IconShape=distinctive  AllPortsSameDT=off  OutDataTypeStr=boolean
  Bus Selector : BusSelector  OutputSignals=signal1,signal2,signal3
  GenericMonitoring2 : Stateflow chart  TreatAsAtomicUnit=on
  Logical Operator1 : Logic  Operator=XOR  AllPortsSameDT=off  OutDataTypeStr=boolean
  Logical Operator2 : Logic  Operator=XOR  AllPortsSameDT=off  OutDataTypeStr=boolean
  Logical Operator3 : Logic  Operator=NOT  AllPortsSameDT=off  OutDataTypeStr=boolean
  Logical Operator4 : Logic  Operator=NOT  AllPortsSameDT=off  OutDataTypeStr=boolean
  Switch : Switch  Criteria=u2 > Threshold
  Switch1 : Switch  Criteria=u2 > Threshold
  Switch2 : Switch  Criteria=u2 > Threshold
  Signal : Outport  OutDataTypeStr=boolean
  Anomaly : Outport  Port=2  OutDataTypeStr=boolean
  wires:
  Bus Selector/1 -> GenericMonitoring2/1(Channel1), Logical Operator1/1, Switch1/1, Switch/1, AND/1  "<signal1>"
  Bus Selector/2 -> AND/2, GenericMonitoring2/2(Channel2), Logical Operator1/2, Logical Operator2/1, Switch2/1  "<signal2>"
  Bus Selector/3 -> AND/3, GenericMonitoring2/3(Channel3), Logical Operator2/2, Switch2/3  "<signal3>"
  In1/1 -> Bus Selector/1
  AND/1 -> Switch/2
  GenericMonitoring2/1(anomaly) -> Anomaly/1
  Switch/1 -> Signal/1
  Logical Operator4/1 -> Switch1/2
  Logical Operator2/1 -> Logical Operator3/1
  Switch2/1 -> Switch1/3
  Switch1/1 -> Switch/3
  Logical Operator3/1 -> Switch2/2
  Logical Operator1/1 -> Logical Operator4/1

== system LGS_allFaultStuffDeleted/Digital Part/Computing module1/GenericMonitoring15 ==
  In1 : Inport
  AND : Logic  Inputs=3  IconShape=distinctive  AllPortsSameDT=off  OutDataTypeStr=boolean
  Bus Selector : BusSelector  OutputSignals=signal1,signal2,signal3
  GenericMonitoring2 : Stateflow chart  TreatAsAtomicUnit=on
  Logical Operator1 : Logic  Operator=XOR  AllPortsSameDT=off  OutDataTypeStr=boolean
  Logical Operator2 : Logic  Operator=XOR  AllPortsSameDT=off  OutDataTypeStr=boolean
  Logical Operator3 : Logic  Operator=NOT  AllPortsSameDT=off  OutDataTypeStr=boolean
  Logical Operator4 : Logic  Operator=NOT  AllPortsSameDT=off  OutDataTypeStr=boolean
  Switch : Switch  Criteria=u2 > Threshold
  Switch1 : Switch  Criteria=u2 > Threshold
  Switch2 : Switch  Criteria=u2 > Threshold
  Signal : Outport  OutDataTypeStr=boolean
  Anomaly : Outport  Port=2  OutDataTypeStr=boolean
  wires:
  Bus Selector/1 -> GenericMonitoring2/1(Channel1), Logical Operator1/1, Switch1/1, Switch/1, AND/1  "<signal1>"
  Bus Selector/2 -> AND/2, GenericMonitoring2/2(Channel2), Logical Operator1/2, Logical Operator2/1, Switch2/1  "<signal2>"
  Bus Selector/3 -> AND/3, GenericMonitoring2/3(Channel3), Logical Operator2/2, Switch2/3  "<signal3>"
  In1/1 -> Bus Selector/1
  AND/1 -> Switch/2
  GenericMonitoring2/1(anomaly) -> Anomaly/1
  Switch/1 -> Signal/1
  Logical Operator4/1 -> Switch1/2
  Logical Operator2/1 -> Logical Operator3/1
  Switch2/1 -> Switch1/3
  Switch1/1 -> Switch/3
  Logical Operator3/1 -> Switch2/2
  Logical Operator1/1 -> Logical Operator4/1

== system LGS_allFaultStuffDeleted/Digital Part/Computing module1/GenericMonitoring16 ==
  In1 : Inport
  AND : Logic  Inputs=3  IconShape=distinctive  AllPortsSameDT=off  OutDataTypeStr=boolean
  Bus Selector : BusSelector  OutputSignals=signal1,signal2,signal3
  GenericMonitoring2 : Stateflow chart  TreatAsAtomicUnit=on
  Logical Operator1 : Logic  Operator=XOR  AllPortsSameDT=off  OutDataTypeStr=boolean
  Logical Operator2 : Logic  Operator=XOR  AllPortsSameDT=off  OutDataTypeStr=boolean
  Logical Operator3 : Logic  Operator=NOT  AllPortsSameDT=off  OutDataTypeStr=boolean
  Logical Operator4 : Logic  Operator=NOT  AllPortsSameDT=off  OutDataTypeStr=boolean
  Switch : Switch  Criteria=u2 > Threshold
  Switch1 : Switch  Criteria=u2 > Threshold
  Switch2 : Switch  Criteria=u2 > Threshold
  Signal : Outport  OutDataTypeStr=boolean
  Anomaly : Outport  Port=2  OutDataTypeStr=boolean
  wires:
  Bus Selector/1 -> GenericMonitoring2/1(Channel1), Logical Operator1/1, Switch1/1, Switch/1, AND/1  "<signal1>"
  Bus Selector/2 -> AND/2, GenericMonitoring2/2(Channel2), Logical Operator1/2, Logical Operator2/1, Switch2/1  "<signal2>"
  Bus Selector/3 -> AND/3, GenericMonitoring2/3(Channel3), Logical Operator2/2, Switch2/3  "<signal3>"
  In1/1 -> Bus Selector/1
  AND/1 -> Switch/2
  GenericMonitoring2/1(anomaly) -> Anomaly/1
  Switch/1 -> Signal/1
  Logical Operator4/1 -> Switch1/2
  Logical Operator2/1 -> Logical Operator3/1
  Switch2/1 -> Switch1/3
  Switch1/1 -> Switch/3
  Logical Operator3/1 -> Switch2/2
  Logical Operator1/1 -> Logical Operator4/1

== system LGS_allFaultStuffDeleted/Digital Part/Computing module1/GenericMonitoring17 ==
  In1 : Inport
  AND : Logic  Inputs=3  IconShape=distinctive  AllPortsSameDT=off  OutDataTypeStr=boolean
  Bus Selector : BusSelector  OutputSignals=signal1,signal2,signal3
  GenericMonitoring2 : Stateflow chart  TreatAsAtomicUnit=on
  Logical Operator1 : Logic  Operator=XOR  AllPortsSameDT=off  OutDataTypeStr=boolean
  Logical Operator2 : Logic  Operator=XOR  AllPortsSameDT=off  OutDataTypeStr=boolean
  Logical Operator3 : Logic  Operator=NOT  AllPortsSameDT=off  OutDataTypeStr=boolean
  Logical Operator4 : Logic  Operator=NOT  AllPortsSameDT=off  OutDataTypeStr=boolean
  Switch : Switch  Criteria=u2 > Threshold
  Switch1 : Switch  Criteria=u2 > Threshold
  Switch2 : Switch  Criteria=u2 > Threshold
  Signal : Outport  OutDataTypeStr=boolean
  Anomaly : Outport  Port=2  OutDataTypeStr=boolean
  wires:
  Bus Selector/1 -> GenericMonitoring2/1(Channel1), Logical Operator1/1, Switch1/1, Switch/1, AND/1  "<signal1>"
  Bus Selector/2 -> AND/2, GenericMonitoring2/2(Channel2), Logical Operator1/2, Logical Operator2/1, Switch2/1  "<signal2>"
  Bus Selector/3 -> AND/3, GenericMonitoring2/3(Channel3), Logical Operator2/2, Switch2/3  "<signal3>"
  In1/1 -> Bus Selector/1
  AND/1 -> Switch/2
  GenericMonitoring2/1(anomaly) -> Anomaly/1
  Switch/1 -> Signal/1
  Logical Operator4/1 -> Switch1/2
  Logical Operator2/1 -> Logical Operator3/1
  Switch2/1 -> Switch1/3
  Switch1/1 -> Switch/3
  Logical Operator3/1 -> Switch2/2
  Logical Operator1/1 -> Logical Operator4/1

== system LGS_allFaultStuffDeleted/Digital Part/Computing module1/GenericMonitoring2 ==
  In1 : Inport
  AND : Logic  Inputs=3  IconShape=distinctive  AllPortsSameDT=off  OutDataTypeStr=boolean
  Bus Selector : BusSelector  OutputSignals=signal1,signal2,signal3
  GenericMonitoring2 : Stateflow chart  TreatAsAtomicUnit=on
  Logical Operator1 : Logic  Operator=XOR  AllPortsSameDT=off  OutDataTypeStr=boolean
  Logical Operator2 : Logic  Operator=XOR  AllPortsSameDT=off  OutDataTypeStr=boolean
  Logical Operator3 : Logic  Operator=NOT  AllPortsSameDT=off  OutDataTypeStr=boolean
  Logical Operator4 : Logic  Operator=NOT  AllPortsSameDT=off  OutDataTypeStr=boolean
  Switch : Switch  Criteria=u2 > Threshold
  Switch1 : Switch  Criteria=u2 > Threshold
  Switch2 : Switch  Criteria=u2 > Threshold
  Signal : Outport  OutDataTypeStr=boolean
  Anomaly : Outport  Port=2  OutDataTypeStr=boolean
  wires:
  Bus Selector/1 -> GenericMonitoring2/1(Channel1), Logical Operator1/1, Switch1/1, Switch/1, AND/1  "<signal1>"
  Bus Selector/2 -> AND/2, GenericMonitoring2/2(Channel2), Logical Operator1/2, Logical Operator2/1, Switch2/1  "<signal2>"
  Bus Selector/3 -> AND/3, GenericMonitoring2/3(Channel3), Logical Operator2/2, Switch2/3  "<signal3>"
  In1/1 -> Bus Selector/1
  AND/1 -> Switch/2
  GenericMonitoring2/1(anomaly) -> Anomaly/1
  Switch/1 -> Signal/1
  Logical Operator4/1 -> Switch1/2
  Logical Operator2/1 -> Logical Operator3/1
  Switch2/1 -> Switch1/3
  Switch1/1 -> Switch/3
  Logical Operator3/1 -> Switch2/2
  Logical Operator1/1 -> Logical Operator4/1

== system LGS_allFaultStuffDeleted/Digital Part/Computing module1/GenericMonitoring3 ==
  In1 : Inport
  AND : Logic  Inputs=3  IconShape=distinctive  AllPortsSameDT=off  OutDataTypeStr=boolean
  Bus Selector : BusSelector  OutputSignals=signal1,signal2,signal3
  GenericMonitoring2 : Stateflow chart  TreatAsAtomicUnit=on
  Logical Operator1 : Logic  Operator=XOR  AllPortsSameDT=off  OutDataTypeStr=boolean
  Logical Operator2 : Logic  Operator=XOR  AllPortsSameDT=off  OutDataTypeStr=boolean
  Logical Operator3 : Logic  Operator=NOT  AllPortsSameDT=off  OutDataTypeStr=boolean
  Logical Operator4 : Logic  Operator=NOT  AllPortsSameDT=off  OutDataTypeStr=boolean
  Switch : Switch  Criteria=u2 > Threshold
  Switch1 : Switch  Criteria=u2 > Threshold
  Switch2 : Switch  Criteria=u2 > Threshold
  Signal : Outport  OutDataTypeStr=boolean
  Anomaly : Outport  Port=2  OutDataTypeStr=boolean
  wires:
  Bus Selector/1 -> GenericMonitoring2/1(Channel1), Logical Operator1/1, Switch1/1, Switch/1, AND/1  "<signal1>"
  Bus Selector/2 -> AND/2, GenericMonitoring2/2(Channel2), Logical Operator1/2, Logical Operator2/1, Switch2/1  "<signal2>"
  Bus Selector/3 -> AND/3, GenericMonitoring2/3(Channel3), Logical Operator2/2, Switch2/3  "<signal3>"
  In1/1 -> Bus Selector/1
  AND/1 -> Switch/2
  GenericMonitoring2/1(anomaly) -> Anomaly/1
  Switch/1 -> Signal/1
  Logical Operator4/1 -> Switch1/2
  Logical Operator2/1 -> Logical Operator3/1
  Switch2/1 -> Switch1/3
  Switch1/1 -> Switch/3
  Logical Operator3/1 -> Switch2/2
  Logical Operator1/1 -> Logical Operator4/1
